simulink model "Dynamic_Nonlinear_BicycleModel"  (R2024b)
settings: Solver=ode8  StartTime=0.0  StopTime=100  FixedStep=0.001  RelTol=1e-3
settings Model: Creator=leandertenbarge  LastModifiedBy=leandertenbarge
settings OptimizationCC: OptimizeBlockIOStorage=off  OptimizeDataStoreBuffers=off  BusAssignmentInplaceUpdate=off
settings DebuggingCC: SFUnexpectedBacktrackingDiag=warning  SFNoUnconditionalDefaultTransitionDiag=warning
settings RTWCC: GenCodeOnly=on  GenerateReport=on  BuildConfiguration=Debug  LaunchReport=on
settings CodeAppCC: ForceParamTrailComments=on  MATLABSourceComments=on  EnableCustomComments=on
settings GRTTargetCC: CombineSignalStateStructs=on  SupportVariableSizeSignals=on  MultiInstanceErrorCode=Warning

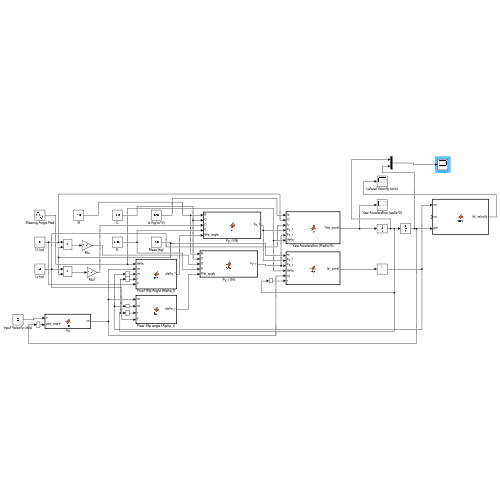
[thumbnail: Simulink's stored preview of the top-level diagram]
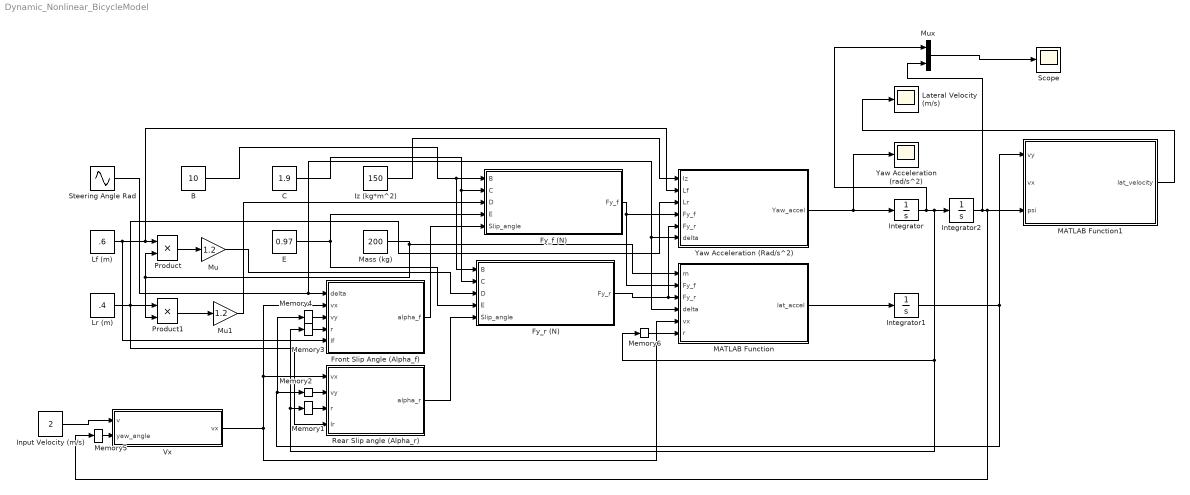
== system Dynamic_Nonlinear_BicycleModel ==
  B : Constant  Value=10
  C : Constant  Value=1.9
  E : Constant  Value=0.97
  Front Slip Angle (Alpha_f) : MATLAB Function  TreatAsAtomicUnit=on
  Fy_f (N) : MATLAB Function  TreatAsAtomicUnit=on
  Fy_r (N) : MATLAB Function  TreatAsAtomicUnit=on
  Input Velocity (m/s) : Constant  Value=2
  Integrator : Integrator
  Integrator1 : Integrator  InitialCondition=0.001
  Integrator2 : Integrator
  Iz (kg*m^2) : Constant  Value=150
  Lateral Velocity (m/s) : Scope
  Lf (m) : Constant  Value=.6
  Lr (m) : Constant  Value=.4
  MATLAB Function : MATLAB Function  TreatAsAtomicUnit=on
  MATLAB Function1 : MATLAB Function  TreatAsAtomicUnit=on
  Mass (kg) : Constant  Value=200
  Memory{1..6} (6 alike) : Memory  InheritSampleTime=on
  Mu : Gain  Gain=1.2
  Mu1 : Gain  Gain=1.2
  Mux : Mux  Inputs=2
  Product : Product
  Product1 : Product
  Rear Slip angle (Alpha_r) : MATLAB Function  TreatAsAtomicUnit=on
  Scope : Scope
  Steering Angle Rad : Sin  Amplitude=0.1  Frequency=.5  SampleTime=0
  Vx : MATLAB Function  TreatAsAtomicUnit=on
  Yaw Acceleration (Rad/s^2) : MATLAB Function  TreatAsAtomicUnit=on
  Yaw Acceleration (rad/s^2) : Scope
  wires:
  Yaw Acceleration (Rad/s^2)/1(Yaw_accel) -> Yaw Acceleration (rad/s^2)/1, Integrator/1
  MATLAB Function/1(lat_accel) -> Integrator1/1
  Memory1/1 -> Rear Slip angle (Alpha_r)/3(r)
  Memory2/1 -> Rear Slip angle (Alpha_r)/2(vy)
  Memory4/1 -> Front Slip Angle (Alpha_f)/3(vy)
  Memory3/1 -> Front Slip Angle (Alpha_f)/4(r)
  Memory5/1 -> Vx/2(yaw_angle)
  Integrator/1 -> Mux/1, Memory3/1, Memory1/1, Memory6/1, Integrator2/1
  Memory6/1 -> MATLAB Function/6(r)
  Integrator1/1 -> Memory4/1, Memory2/1, MATLAB Function1/1(vy)
  MATLAB Function1/1(lat_velocity) -> Lateral Velocity (m/s)/1
  Product/1 -> Mu/1
  Mu/1 -> Fy_r (N)/3(D)
  Lf (m)/1 -> Front Slip Angle (Alpha_f)/5(lf), Yaw Acceleration (Rad/s^2)/2(Lf), Product/1
  Mass (kg)/1 -> MATLAB Function/1(m), Product1/2, Product/2
  Lr (m)/1 -> Rear Slip angle (Alpha_r)/4(lr), Yaw Acceleration (Rad/s^2)/3(Lr), Product1/1
  Product1/1 -> Mu1/1
  Mu1/1 -> Fy_f (N)/3(D)
  B/1 -> Fy_f (N)/1(B), Fy_r (N)/1(B)
  C/1 -> Fy_r (N)/2(C), Fy_f (N)/2(C)
  E/1 -> Fy_r (N)/4(E), Fy_f (N)/4(E)
  Rear Slip angle (Alpha_r)/1(alpha_r) -> Fy_r (N)/5(Slip_angle)
  Front Slip Angle (Alpha_f)/1(alpha_f) -> Fy_f (N)/5(Slip_angle)
  Vx/1(vx) -> MATLAB Function/5(vx), Front Slip Angle (Alpha_f)/2(vx), Rear Slip angle (Alpha_r)/1(vx)
  Input Velocity (m/s)/1 -> Vx/1(v)
  Steering Angle Rad/1 -> MATLAB Function/4(delta), Yaw Acceleration (Rad/s^2)/6(delta), Front Slip Angle (Alpha_f)/1(delta)
  Fy_f (N)/1(Fy_f) -> Yaw Acceleration (Rad/s^2)/4(Fy_f), MATLAB Function/2(Fy_f)
  Fy_r (N)/1(Fy_r) -> Yaw Acceleration (Rad/s^2)/5(Fy_r), MATLAB Function/3(Fy_r)
  Iz (kg*m^2)/1 -> Yaw Acceleration (Rad/s^2)/1(Iz)
  Integrator2/1 -> Mux/2, Memory5/1, MATLAB Function1/3(psi)
  Mux/1 -> Scope/1

== matlab function Dynamic_Nonlinear_BicycleModel/Rear Slip angle (Alpha_r) ==
  data: alpha_r output; vx input; vy input; r input; lr input
function alpha_r = fcn(vx,vy,r,lr)

alpha_r = atan(vy-lr*r)/(vx);

== matlab function Dynamic_Nonlinear_BicycleModel/Front Slip Angle (Alpha_f) ==
  data: delta input; alpha_f output; vx input; vy input; r input; lf input
function alpha_f = fcn(delta,vx,vy,r,lf)

alpha_f = delta - atan(vy+lf*r)/(vx);

== matlab function Dynamic_Nonlinear_BicycleModel/Vx ==
  data: v input; vx output; yaw_angle input
function vx = fcn(v,yaw_angle)
%#codegen

vx = v*cos(yaw_angle);

== matlab function Dynamic_Nonlinear_BicycleModel/Fy_f (N) ==
  data: B input; Fy_f output; C input; D input; E input; Slip_angle input
function Fy_f  = fcn(B,C,D,E,Slip_angle)

Fy_f = D*sin(C*atan(B*Slip_angle- E*(B*Slip_angle- atan(B*Slip_angle))));

== matlab function Dynamic_Nonlinear_BicycleModel/Fy_r (N) ==
  data: B input; Fy_r output; C input; D input; E input; Slip_angle input
function Fy_r  = fcn(B,C,D,E,Slip_angle)

Fy_r = D*sin(C*atan(B*Slip_angle- E*(B*Slip_angle- atan(B*Slip_angle))));

== matlab function Dynamic_Nonlinear_BicycleModel/Yaw Acceleration (Rad//s^2) ==
  data: Iz input; Yaw_accel output; Lf input; Lr input; Fy_f input; Fy_r input; delta input
function Yaw_accel = fcn(Iz,Lf,Lr,Fy_f,Fy_r,delta)
%#codegen

Yaw_accel = (1/Iz)*(Lf*Fy_f*cos(delta)-Lr*Fy_r);

== matlab function Dynamic_Nonlinear_BicycleModel/MATLAB Function ==
  data: m input; lat_accel output; Fy_f input; Fy_r input; delta input; vx input; r input
function lat_accel = fcn(m,Fy_f, Fy_r,delta,vx,r)

lat_accel = (1/m)*(Fy_f*cos(delta+Fy_r)-vx*r);

== matlab function Dynamic_Nonlinear_BicycleModel/MATLAB Function1 ==
  data: vy input; lat_velocity output; vx input; psi input
function lat_velocity = fcn(vy,vx,psi)

lat_velocity = vy*cos(psi)+vx*sin(psi);
